simulink model "ADMM_consensus"  (R2022b)
settings: Solver=VariableStepAuto  StartTime=0.0  StopTime=10.0  RelTol=1e-3
values from neighbouring files (symbols this model uses):
  c = scaled_standard_constants    [comparision.m]
settings Model: Creator=is123  LastModifiedBy=is123

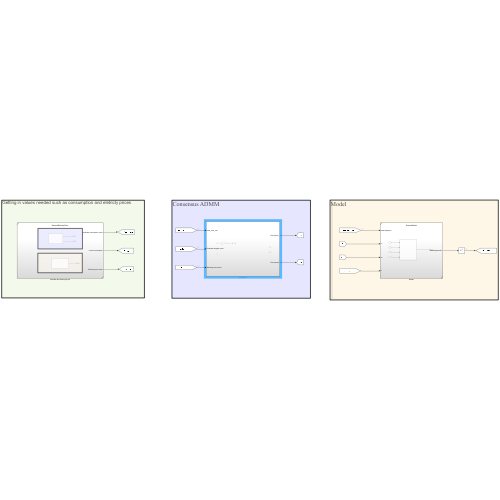
[thumbnail: Simulink's stored preview of the top-level diagram]
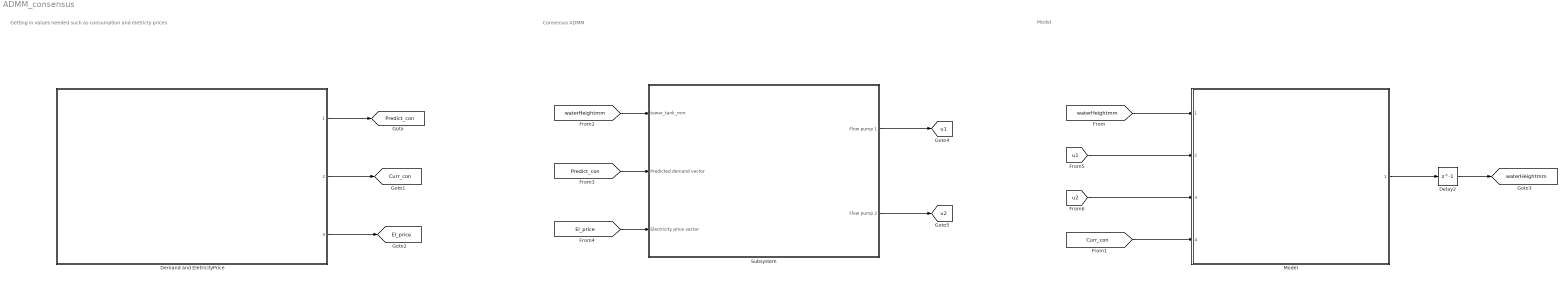
== system ADMM_consensus ==
  note: Getting in values needed such as consumption and eletricty prices
  note: Consensus ADMM
  note: Model
  Delay2 : Delay  DelayLength=1  InitialCondition=c.V/c.At*1e3
  Demand and EletricityPrice : Subsystem  ReferencedSubsystem=DemandEletricityPrice
  Model : Subsystem  ReferencedSubsystem=SimulinkModel
  Subsystem : Subsystem
  tag scope: Curr_con=global, El_price=global, Predict_con=global, u1=global, u2=global, waterHeightmm=global
  wires:
  Demand and EletricityPrice/1 -> [Predict_con]
  Demand and EletricityPrice/2 -> [Curr_con]
  Demand and EletricityPrice/3 -> [El_price]
  Model/1 -> Delay2/1
  Delay2/1 -> [waterHeightmm]
  [waterHeightmm] -> Model/1
  [Curr_con] -> Model/4
  [waterHeightmm] -> Subsystem/1(tower_tank_mm)
  [Predict_con] -> Subsystem/2(Predicted demand vector)
  [El_price] -> Subsystem/3(Electricity price vector)
  Subsystem/1(Flow pump 1) -> [u1]
  Subsystem/2(Flow pump 2) -> [u2]
  [u1] -> Model/2
  [u2] -> Model/3

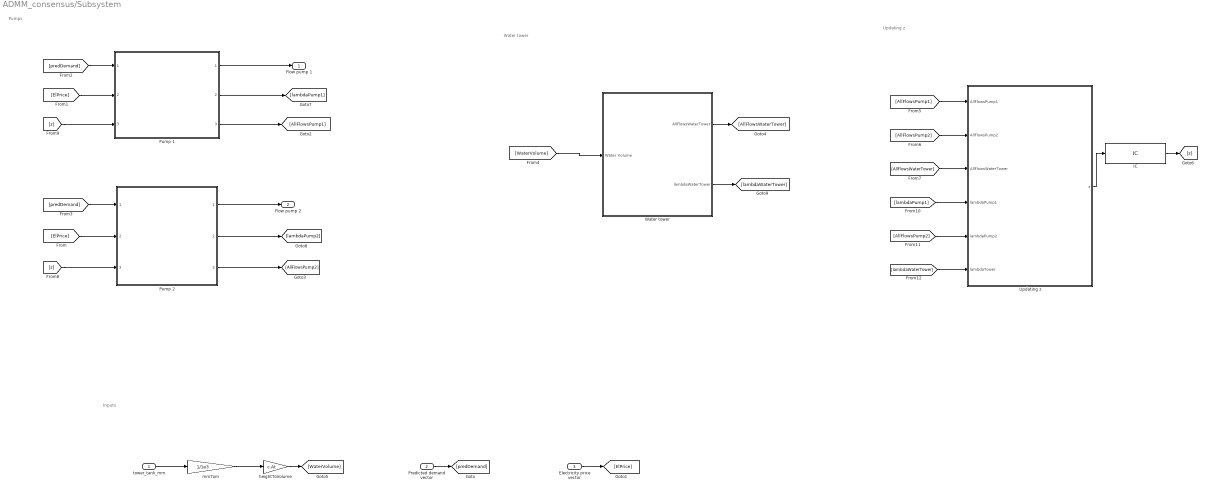
== system ADMM_consensus/Subsystem ==
  note: Updating z
  note: Water tower
  note: Pumps
  note: Inputs
  tower_tank_mm : Inport
  Predicted demand vector : Inport  Port=2
  Electricity price vector : Inport  Port=3
  IC : InitialCondition  Value=zeros(c.Nu*c.Nc,1)
  "Pump 1 " : Subsystem  ReferencedSubsystem=consensusPump  n_unit=1
  Pump 2 : Subsystem  ReferencedSubsystem=consensusPump  n_unit=2
  Updating z : Subsystem
  Water tower : Subsystem
  heightToVolume : Gain  Gain=c.At
  mmTom : Gain  Gain=1/1e3
  Flow pump 1 : Outport
  Flow pump 2 : Outport  Port=2
  wires:
  mmTom/1 -> heightToVolume/1
  tower_tank_mm/1 -> mmTom/1
  "Pump 1 "/1 -> Flow pump 1/1
  Pump 2/1 -> Flow pump 2/1
  Predicted demand vector/1 -> [predDemand]
  Electricity price vector/1 -> [ElPrice]
  [ElPrice] -> Pump 2/2
  [ElPrice] -> "Pump 1 "/2
  [predDemand] -> "Pump 1 "/1
  [predDemand] -> Pump 2/1
  "Pump 1 "/3 -> [AllFlowsPump1]
  Pump 2/3 -> [AllFlowsPump2]
  Water tower/1(AllFlowsWaterTower) -> [AllFlowsWaterTower]
  heightToVolume/1 -> [WaterVolume]
  [WaterVolume] -> Water tower/1(Water Volume)
  [AllFlowsPump1] -> Updating z/1(AllFlowsPump1)
  [AllFlowsPump2] -> Updating z/2(AllFlowsPump2)
  [AllFlowsWaterTower] -> Updating z/3(AllFlowsWaterTower)
  Updating z/1(z) -> IC/1
  [z] -> Pump 2/3
  [z] -> "Pump 1 "/3
  IC/1 -> [z]
  [lambdaPump1] -> Updating z/4(lambdaPump1)
  "Pump 1 "/2 -> [lambdaPump1]
  Pump 2/2 -> [lambdaPump2]
  [AllFlowsPump2] -> Updating z/5(lambdaPump2)
  Water tower/2(lambdaWaterTower) -> [lambdaWaterTower]
  [lambdaWaterTower] -> Updating z/6(lambdaTower)

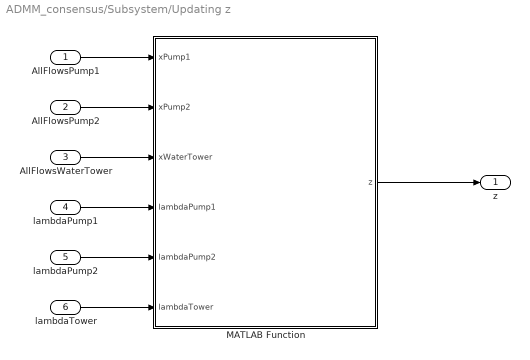
== system ADMM_consensus/Subsystem/Updating z ==
  AllFlowsPump1 : Inport
  AllFlowsPump2 : Inport  Port=2
  AllFlowsWaterTower : Inport  Port=3
  lambdaPump1 : Inport  Port=4
  lambdaPump2 : Inport  Port=5
  lambdaTower : Inport  Port=6
  MATLAB Function : MATLAB Function  TreatAsAtomicUnit=on  SystemSampleTime=3600/c.AccTime
  z : Outport
  wires:
  MATLAB Function/1(z) -> z/1
  AllFlowsPump1/1 -> MATLAB Function/1(xPump1)
  AllFlowsPump2/1 -> MATLAB Function/2(xPump2)
  AllFlowsWaterTower/1 -> MATLAB Function/3(xWaterTower)
  lambdaPump1/1 -> MATLAB Function/4(lambdaPump1)
  lambdaPump2/1 -> MATLAB Function/5(lambdaPump2)
  lambdaTower/1 -> MATLAB Function/6(lambdaTower)

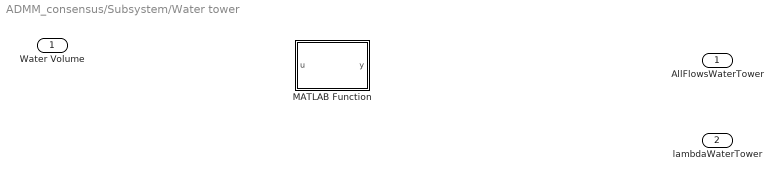
== system ADMM_consensus/Subsystem/Water tower ==
  Water Volume : Inport
  MATLAB Function : MATLAB Function  TreatAsAtomicUnit=on  SystemSampleTime=3600/c.AccTime
  AllFlowsWaterTower : Outport
  lambdaWaterTower : Outport  Port=2

== matlab function ADMM_consensus/Subsystem/Updating z/MATLAB Function ==
  data: xPump1 input; xPump2 input; z output; xWaterTower input; lambdaPump1 input; lambdaPump2 input; lambdaTower input
function z = updateZ(xPump1,xPump2,xWaterTower,lambdaPump1,lambdaPump2,lambdaTower)
%Here it is desired to determine the next value of z, 
%Loading in standard contants
c=scaled_standard_constants; 

%Defining the size of the output
z=zeros(c.Nu*c.Nc,1); 

%Making is of the term in the sum: 
zPump1=1/c.Nu*(xPump1+1/rho*lambdaPump1); 

zPump2=1/c.Nu*(xPump2+1/rho*lambdaPump2);

zWaterTower=1/c.Nu*(xWaterTower+1/rho*lambdaTower);

%Addning them up to get the output:
z=zPump1+zPump2+zWaterTower;

== matlab function ADMM_consensus/Subsystem/Water tower/MATLAB Function ==
  data: u input; y output
function y = fcn(u)

y = u;
